simulink model "two_dof_system_state_space"  (R2019a)
settings: Solver=VariableStepAuto  StartTime=0.0  StopTime=5  RelTol=1e-3
values from neighbouring files (symbols this model uses):
  A = [c_11,c_21,c_31,c_41;c_12,c_22,c_32,c_42;l_1*c_11,l_2*c_21,l_3*c_31,l_4*c_41;l_1*c_12,l_2*c_22,l_3*c_32,l_4*c_42]    [cost_function.m]    (also in fourier_transform_two_dof_free.m; two_dof_system_free_oscillations.m)
  w_0 = [x_0;p_0;x_dot_0;p_dot_0]    [cost_function.m]    (also in fourier_transform_two_dof_free.m; two_dof_system_free_oscillations.m)
settings Model: Creator=HP  LastModifiedBy=HP

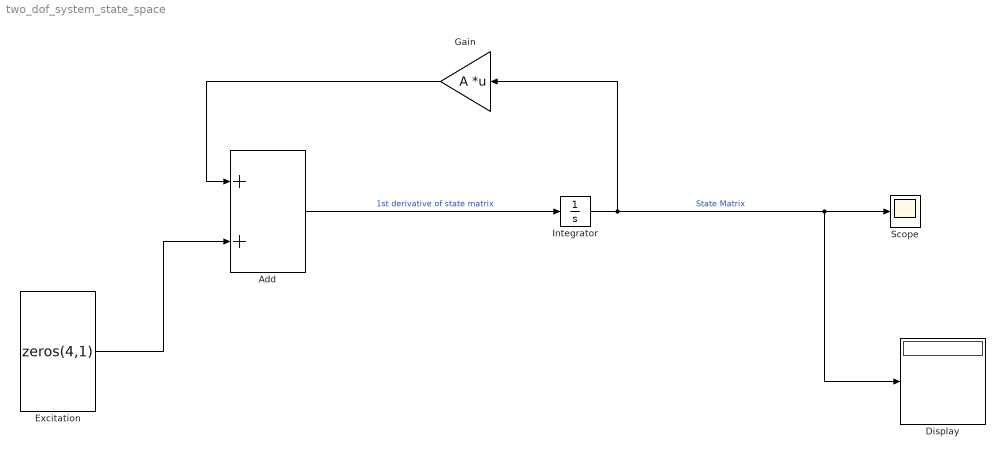
== system two_dof_system_state_space ==
  Add : Sum
  Display : Display
  "Excitation " : Constant  Value=zeros(4,1)
  Gain : Gain  Gain=A  Multiplication=Matrix(K*u)
  Integrator : Integrator  InitialCondition=w_0
  Scope : Scope
  wires:
  Add/1 -> Integrator/1  "1st derivative of state matrix"
  Integrator/1 -> Gain/1, Display/1, Scope/1  "State Matrix"
  Gain/1 -> Add/1
  "Excitation "/1 -> Add/2
